simulink model "orbitalTransferSim"  (R2020b)
settings: Solver=ode45  StartTime=0.0  StopTime=24*3600*3  RelTol=1e-12
values from neighbouring files (symbols this model uses):
  IC = [-Xi 0 0        0 -v 0         M]    [main.m]
  ISP = 2100*0.99    (= 2079)    [main.m]
  mu = 3.986005*10^5    (= 398600.5)    [main.m]
  thrust = 5    [main.m]
  v_des = sqrt(mu/r_des)    [main.m]
libraries: simulink_extras x2
settings Model: Creator=mach1337  LastModifiedBy=mach1337

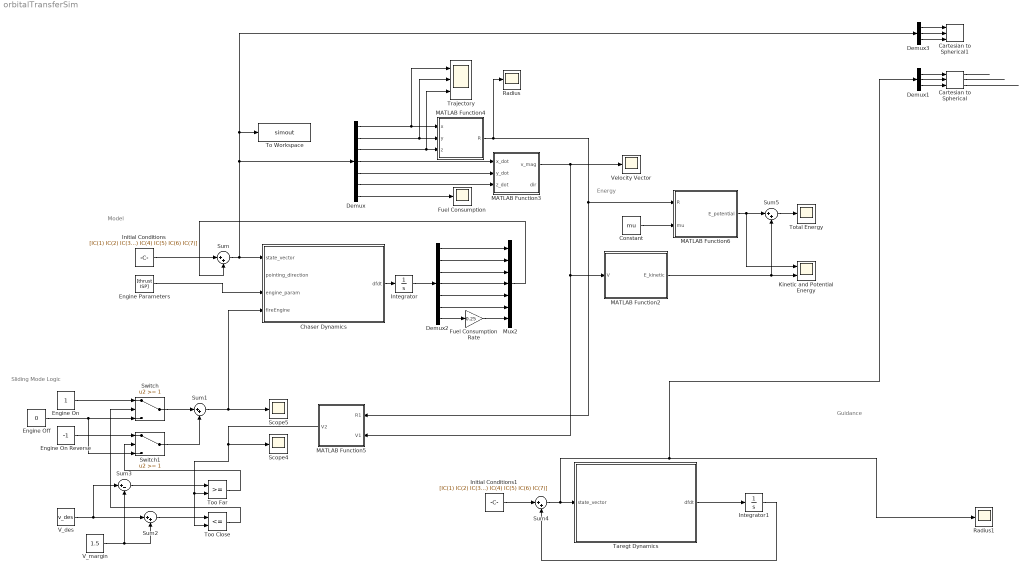
== system orbitalTransferSim ==
  note: Sliding Mode Logic
  note: Energy
  note: Model
  note: Guidance
  Cartesian to Spherical : simulink_extras/Transformations/Cartesian to Spherical
      settings: SourceProductBaseCode=SL
  Cartesian to Spherical1 : simulink_extras/Transformations/Cartesian to Spherical
      settings: SourceProductBaseCode=SL
  Chaser Dynamics : MATLAB Function  TreatAsAtomicUnit=on
  Constant : Constant  Value=mu
  Demux : Demux  Outputs=7
  Demux1 : Demux  Outputs=3
  Demux2 : Demux  Outputs=7
  Demux3 : Demux  Outputs=3
  Engine Off : Constant  Value=0  OutDataTypeStr=Inherit: Inherit via back propagation
  Engine On : Constant
  Engine On Reverse : Constant  Value=-1
  Engine Parameters : Constant  Value=[thrust ISP]
  Fuel Consumption : Scope
  Fuel Consumption Rate : Gain  Gain=0.25
  Initial Conditions : Constant  Value=[IC(1) IC(2) IC(3) IC(4) IC(5) IC(6) IC(7)]
  Initial Conditions1 : Constant  Value=[IC(1) IC(2) IC(3) IC(4) IC(5) IC(6) IC(7)]
  Integrator : Integrator
  Integrator1 : Integrator
  Kinetic and Potential Energy : Scope  NumInputPorts=2
  MATLAB Function2 : MATLAB Function  TreatAsAtomicUnit=on
  MATLAB Function3 : MATLAB Function  TreatAsAtomicUnit=on
  MATLAB Function4 : MATLAB Function  TreatAsAtomicUnit=on
  MATLAB Function5 : MATLAB Function  TreatAsAtomicUnit=on
  MATLAB Function6 : MATLAB Function  TreatAsAtomicUnit=on
  Mux2 : Mux  Inputs=7
  Radius : Scope
  Radius1 : Scope
  Scope4 : Scope
  Scope5 : Scope
  Sum{,1..2,4..5} (5 alike) : Sum  Inputs=|++
  Sum3 : Sum  Inputs=|+-
  Switch : Switch  Threshold=1
  Switch1 : Switch  Threshold=1
  Taregt Dynamics : MATLAB Function  TreatAsAtomicUnit=on
  To Workspace : ToWorkspace  VariableName=simout  SaveFormat=Timeseries  SampleTime=-1
  Too Close : RelationalOperator  Operator=<=  OutDataTypeStr=boolean  RndMeth=Simplest
  Too Far : RelationalOperator  OutDataTypeStr=boolean  RndMeth=Simplest
  Total Energy : Scope
  Trajectory : Scope  NumInputPorts=3
  V_des : Constant  Value=v_des
  V_margin : Constant  Value=1.5
  Velocity Vector : Scope
  wires:
  Engine Parameters/1 -> Chaser Dynamics/3(engine_param)
  Chaser Dynamics/1(dfdt) -> Integrator/1
  Initial Conditions/1 -> Sum/1
  Sum/1 -> Demux3/1, To Workspace/1, Demux/1, Chaser Dynamics/1(state_vector)
  Demux/4 -> MATLAB Function3/1(x_dot)
  Demux/5 -> MATLAB Function3/2(y_dot)
  Demux/6 -> MATLAB Function3/3(z_dot)
  Demux/7 -> Fuel Consumption/1
  Integrator/1 -> Demux2/1
  Engine On/1 -> Switch/1
  MATLAB Function3/1(v_mag) -> Velocity Vector/1, MATLAB Function2/1(V), MATLAB Function5/2(V1)
  MATLAB Function5/1(V2) -> Too Close/2, Too Far/2, Scope4/1
  Engine Off/1 -> Switch1/3, Switch/3
  Engine On Reverse/1 -> Switch1/1
  Switch/1 -> Sum1/1
  Switch1/1 -> Sum1/2
  V_des/1 -> Sum3/1, Sum2/1
  V_margin/1 -> Sum2/2, Sum3/2
  Sum3/1 -> Too Far/1
  Sum2/1 -> Too Close/1
  Too Far/1 -> Switch1/2
  Too Close/1 -> Switch/2
  Sum1/1 -> Chaser Dynamics/4(fireEngine), Scope5/1
  Demux2/7 -> Fuel Consumption Rate/1
  Fuel Consumption Rate/1 -> Mux2/7
  Demux2/6 -> Mux2/6
  Demux2/5 -> Mux2/5
  Demux2/4 -> Mux2/4
  Demux2/3 -> Mux2/3
  Demux2/2 -> Mux2/2
  Demux2/1 -> Mux2/1
  Mux2/1 -> Sum/2
  MATLAB Function2/1(E_kinetic) -> Kinetic and Potential Energy/2, Sum5/2
  Constant/1 -> MATLAB Function6/2(mu)
  Sum5/1 -> Total Energy/1
  MATLAB Function6/1(E_potential) -> Sum5/1, Kinetic and Potential Energy/1
  Demux/3 -> Trajectory/3, MATLAB Function4/3(z)
  Demux/2 -> Trajectory/2, MATLAB Function4/2(y)
  Demux/1 -> Trajectory/1, MATLAB Function4/1(x)
  Taregt Dynamics/1(dfdt) -> Integrator1/1
  Integrator1/1 -> Sum4/2
  Initial Conditions1/1 -> Sum4/1
  Sum4/1 -> Demux1/1, Radius1/1, Taregt Dynamics/1(state_vector)
  Demux1/1 -> Cartesian to Spherical/1
  Demux1/2 -> Cartesian to Spherical/2
  Demux1/3 -> Cartesian to Spherical/3
  Cartesian to Spherical/3 -> ?
  Cartesian to Spherical/2 -> ?
  Cartesian to Spherical/1 -> ?
  Demux3/3 -> Cartesian to Spherical1/3
  Demux3/2 -> Cartesian to Spherical1/2
  Demux3/1 -> Cartesian to Spherical1/1
  MATLAB Function4/1(R) -> MATLAB Function6/1(R), MATLAB Function5/1(R1), Radius/1
  ? -> Chaser Dynamics/2(pointing_direction)

== matlab function orbitalTransferSim/Taregt Dynamics ==
  data: dfdt output; state_vector input
function dfdt = EOM(state_vector)

    % Constants
    mu=3.986005*10^5;         % [km^3/s^2] 
    g0=9.8066;                % [m/s] gravity

    dfdt = zeros(size(state_vector));
    x     = state_vector(1); % x
    y     = state_vector(2); % y
    z     = state_vector(3); % z
    x_dot = state_vector(4); % dx/dt
    y_dot = state_vector(5); % dy/dt
    z_dot = state_vector(6); % dz/dt

    r=sqrt(x^2+y^2+z^2);

    dfdt(1) = x_dot;
    dfdt(2) = y_dot;
    dfdt(3) = z_dot;
    dfdt(4) = -mu*x/r^3;
    dfdt(5) = -mu*y/r^3;
    dfdt(6) = -mu*z/r^3;

== matlab function orbitalTransferSim/Chaser Dynamics ==
  data: dfdt output; state_vector input; pointing_direction input; engine_param input; fireEngine input
function dfdt = EOM(state_vector, pointing_direction,engine_param, fireEngine)

    % Constants
    mu=3.986005*10^5;         % [km^3/s^2] 
    g0=9.8066;                % [m/s] gravity

    % Engine Parameters
    thrust = engine_param(1); % [N] engine thrust 
    ISP = engine_param(2);    % [s] specific impulse engine

    dfdt = zeros(size(state_vector));
    x     = state_vector(1); % x
    y     = state_vector(2); % y
    z     = state_vector(3); % z
    x_dot = state_vector(4); % dx/dt
    y_dot = state_vector(5); % dy/dt
    z_dot = state_vector(6); % dz/dt
    m     = state_vector(7); % mass

    r=sqrt(x^2+y^2+z^2);

    if fireEngine == 1
        vel = [x_dot y_dot z_dot];
        vel_dir = vel/norm(vel);
        pos = [x y z];
        pos_dir = pos/norm(pos);
        F = (thrust/m)/1000;
        F = F.*pointing_direction;
        %F = F.*pos_dir;
        Fx = F(1);
        Fy = F(2);
        Fz = F(3);
        mass = -thrust/(ISP*g0);
    else
        Fx = 0;
        Fy = 0;
        Fz = 0;
        mass = 0;
    end

    dfdt(1) = x_dot;
    dfdt(2) = y_dot;
    dfdt(3) = z_dot;
    dfdt(4) = -mu*x/r^3 + Fx;
    dfdt(5) = -mu*y/r^3 + Fy;
    dfdt(6) = -mu*z/r^3 + Fz;
    dfdt(7) = mass;

== matlab function orbitalTransferSim/MATLAB Function2 ==
  data: V input; E_kinetic output
function E_kinetic = energy(V)

E_kinetic = V^2/2;

== matlab function orbitalTransferSim/MATLAB Function3 ==
  data: x_dot input; v_mag output; y_dot input; z_dot input; dir output
function [v_mag, dir]= vel(x_dot, y_dot, z_dot)

v = [x_dot, y_dot, z_dot];

dir = v/norm(v);
v_mag = sqrt(x_dot^2 + y_dot^2 + z_dot^2);

== matlab function orbitalTransferSim/MATLAB Function4 ==
  data: x input; R output; y input; z input
function R = fcn(x, y, z)

R = sqrt(x^2 + y^2 + z^2);

== matlab function orbitalTransferSim/MATLAB Function5 ==
  data: R1 input; V2 output; V1 input
function V2 = fcn(R1, V1)

R2 = 35786;% desired orbit
mu = 3.9860e+05;

V2 = sqrt(mu/R1)*(sqrt(2*R2/(R1+R2)) - 1)+V1;

== matlab function orbitalTransferSim/MATLAB Function6 ==
  data: R input; E_potential output; mu input
function E_potential = energy(R, mu)

E_potential = -mu/R;
